simulink model "simulation_pv_parallel"  (R2020b)
settings: Solver=FixedStepAuto  StartTime=0.0  StopTime=sim_length  FixedStep=1  RelTol=1e-3
values from neighbouring files (symbols this model uses):
  air_delay = 0    [analysis.m]    (also in config.m; matlab.mat; workspace.mat)
  air_pulse = (air_time * 100)/period    [analysis.m]    (also in config.m = 25; matlab.mat = 25; workspace.mat = 25)
  efficiency_pv = [0.0206 0.0224 0.0235 0.0258 0.0287 0.0304 0.0361 0.0396 0.0436 0.047 0.0774 0.0866 ... (52 elements, 26x2)]    [matlab.mat]    (also in workspace.mat)
  efficiencybatterydcdc = [0.0136458313659 0.015570408259 0.019337485453 0.0242437613353 0.0298263424578 0.0373938343643 0.0491473380199 0.0560789663375 0.0670656286702 0.0809654995908 0.0941455940195 0.113657997475 ... (56 elements, 28x2)]    [workspace.mat]
  G = [250;500;750;1000]    [lab3_day1.m]    (also in matlab.mat = [250 500 750 1000]; workspace.mat = [250 500 750 1000])
  I = [Impp_250;Impp_500;Impp_750;Impp_1000]    [lab3_day1.m]    (also in matlab.mat = [0.01272 0.02816 0.04153 0.05463]; workspace.mat = [0.01272 0.02816 0.04153 0.05463])
  mc_delay = mic_delay + mic_time    [analysis.m]    (also in config.m = 30; matlab.mat = 30; workspace.mat = 30)
  mc_pulse = (mc_time*100)/period    [analysis.m]    (also in config.m = 5; matlab.mat = 5; workspace.mat = 5)
  methane_delay = air_time    [analysis.m]    (also in config.m = 0; matlab.mat = 0; workspace.mat = 0)
  methane_pulse = (methane_time * 100)/period    [analysis.m]    (also in config.m = 25; matlab.mat = 25; workspace.mat = 25)
  mic_delay = temp_delay + temp_time    [analysis.m]    (also in config.m = 0; matlab.mat = 0; workspace.mat = 0)
  mic_pulse = (mic_time * 100)/period    [analysis.m]    (also in config.m = 10; matlab.mat = 10; workspace.mat = 10)
  period = 240    [analysis.m]    (also in config.m = 120; matlab.mat = 120; workspace.mat = 120)
  temp_delay = methane_delay + methane_time    [analysis.m]    (also in config.m = 0; matlab.mat = 0; workspace.mat = 0)
  temp_pulse = (temp_time *100)/period    [analysis.m]    (also in config.m = 5; matlab.mat = 5; workspace.mat = 5)
  transmit_delay = mc_delay + mc_time    [analysis.m]    (also in config.m = 36; matlab.mat = 36; workspace.mat = 36)
  transmit_pulse = (transmit_time * 100)/period    [analysis.m]    (also in config.m = 20; matlab.mat = 20; workspace.mat = 20)
  V = [Vmpp_250;Vmpp_500;Vmpp_750;Vmpp_1000]    [lab3_day1.m]    (also in matlab.mat = [3.1 3.14 3.15 3.3]; workspace.mat = [3.1 3.14 3.15 3.3])
libraries: simulink x10
settings Model: Creator=sara  LastModifiedBy=Nicolò
settings DataIOCC: ReturnWorkspaceOutputs=off
settings DebuggingCC: ArithmeticOperatorsInVariantConditions=warning
settings SFSimCC: SimUseLocalCustomCode=off  CustomCodeUndefinedFunction=UseInterfaceOnly
settings RTWCC: RTWUseLocalCustomCode=off
settings CodeAppCC: StateflowObjectComments=on

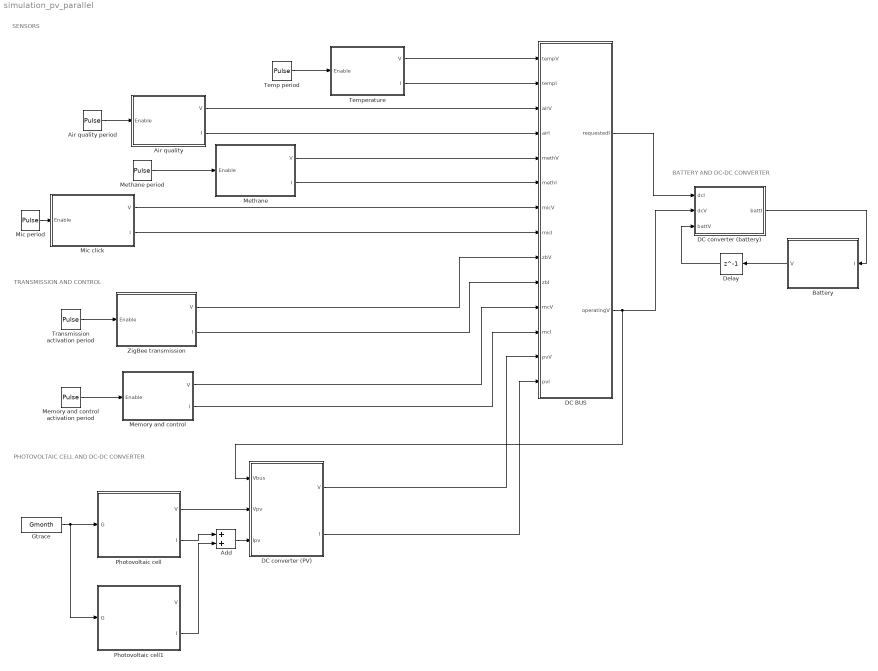
== system simulation_pv_parallel ==
  note: TRANSMISSION AND CONTROL
  note: SENSORS
  note: PHOTOVOLTAIC CELL AND DC-DC CONVERTER
  note: BATTERY AND DC-DC CONVERTER
  Add : Sum
  Air quality : Subsystem
  Air quality period : DiscretePulseGenerator  PulseType=Time based  Period=period  PulseWidth=air_pulse  PhaseDelay=air_delay
  Battery : Subsystem
  DC BUS : Subsystem
  DC converter (PV) : Subsystem
  DC converter (battery) : Subsystem
  Delay : Delay  DelayLength=1  InitialCondition=0
  Gtrace : FromWorkspace  VariableName=Gmonth  OutputAfterFinalValue=Setting to zero
  Memory and control : Subsystem
  Memory and control activation period : DiscretePulseGenerator  PulseType=Time based  Period=period  PulseWidth=mc_pulse  PhaseDelay=mc_delay
  Methane : Subsystem
  Methane period : DiscretePulseGenerator  PulseType=Time based  Period=period  PulseWidth=methane_pulse  PhaseDelay=methane_delay
  Mic period : DiscretePulseGenerator  PulseType=Time based  Period=period  PulseWidth=mic_pulse  PhaseDelay=mic_delay
  Mic click : Subsystem
  Photovoltaic cell : Subsystem
  Photovoltaic cell1 : Subsystem
  Temp period : DiscretePulseGenerator  PulseType=Time based  Period=period  PulseWidth=temp_pulse  PhaseDelay=temp_delay
  Temperature : Subsystem
  Transmission activation period : DiscretePulseGenerator  PulseType=Time based  Period=period  PulseWidth=transmit_pulse  PhaseDelay=transmit_delay
  ZigBee transmission : Subsystem
  wires:
  Gtrace/1 -> Photovoltaic cell1/1(G), Photovoltaic cell/1(G)
  Mic click/2(I) -> DC BUS/8(micI)
  Mic click/1(V) -> DC BUS/7(micV)
  Mic period/1 -> Mic click/1(Enable)
  Air quality period/1 -> Air quality/1(Enable)
  Air quality/1(V) -> DC BUS/3(airV)
  Air quality/2(I) -> DC BUS/4(airI)
  Methane/1(V) -> DC BUS/5(methV)
  Methane period/1 -> Methane/1(Enable)
  Methane/2(I) -> DC BUS/6(methI)
  Temperature/1(V) -> DC BUS/1(tempV)
  Temp period/1 -> Temperature/1(Enable)
  ZigBee transmission/1(V) -> DC BUS/9(zbV)
  Transmission activation period/1 -> ZigBee transmission/1(Enable)
  Temperature/2(I) -> DC BUS/2(tempI)
  Memory and control/1(V) -> DC BUS/11(mcV)
  ZigBee transmission/2(I) -> DC BUS/10(zbI)
  Battery/1(V) -> Delay/1
  DC converter (battery)/1(battI) -> Battery/1(I)
  DC BUS/1(requestedI) -> DC converter (battery)/1(dcI)
  DC BUS/2(operatingV) -> DC converter (PV)/1(Vbus), DC converter (battery)/2(dcV)
  Delay/1 -> DC converter (battery)/3(battV)
  DC converter (PV)/2(I) -> DC BUS/14(pvI)
  DC converter (PV)/1(V) -> DC BUS/13(pvV)
  Memory and control/2(I) -> DC BUS/12(mcI)
  Memory and control activation period/1 -> Memory and control/1(Enable)
  Add/1 -> DC converter (PV)/3(Ipv)
  Photovoltaic cell/2(I) -> Add/1
  Photovoltaic cell1/2(I) -> Add/2
  Photovoltaic cell/1(V) -> DC converter (PV)/2(Vpv)

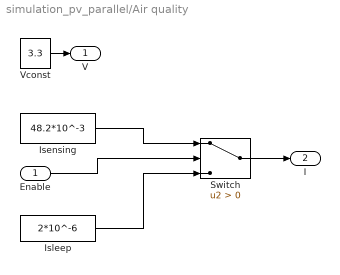
== system simulation_pv_parallel/Air quality ==
  Enable : Inport
  Isensing : Constant  Value=48.2*10^-3
  Isleep : Constant  Value=2*10^-6
  Switch : Switch  Criteria=u2 > Threshold
  Vconst : Constant  Value=3.3
  V : Outport
  I : Outport  Port=2
  wires:
  Enable/1 -> Switch/2
  Isleep/1 -> Switch/3
  Vconst/1 -> V/1
  Isensing/1 -> Switch/1
  Switch/1 -> I/1

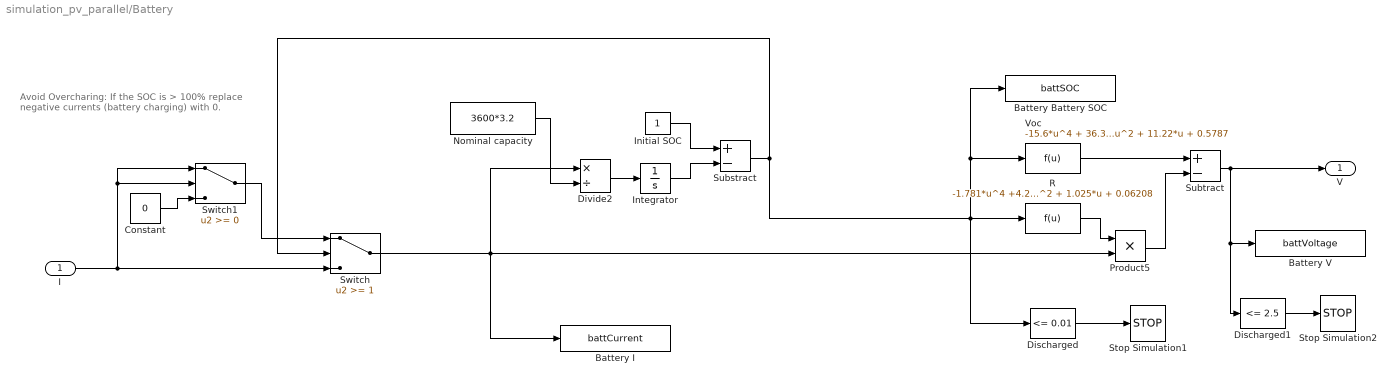
== system simulation_pv_parallel/Battery ==
  note: Avoid Overcharing:
      | If the SOC is > 100% replace negative currents (battery charging) with 0.
  I : Inport
  Battery Battery SOC : ToWorkspace  VariableName=battSOC  SampleTime=-1
  Battery I : ToWorkspace  VariableName=battCurrent  SampleTime=-1
  Battery V : ToWorkspace  VariableName=battVoltage  SampleTime=-1
  Constant : Constant  Value=0
  Discharged : simulink/Logic and Bit Operations/Compare To Constant  relop=<=  const=0.01  OutDataTypeStr=boolean  ZeroCross=off
  Discharged1 : simulink/Logic and Bit Operations/Compare To Constant  relop=<=  const=2.5  OutDataTypeStr=boolean  ZeroCross=off
  Divide2 : Product  Inputs=*/
  Initial SOC : Constant
  Integrator : Integrator
  Nominal capacity : Constant  Value=3600*3.2
  Product5 : Product  RndMeth=Zero
  R : Fcn  Expr=-1.781*u^4 +4.222*u^3 -3.401*u^2 + 1.025*u + 0.06208
  Stop Simulation1 : Stop
  Stop Simulation2 : Stop
  Substract : Sum  Inputs=+-
  Subtract : Sum  Inputs=+-
  Switch : Switch  Threshold=1
  Switch1 : Switch
  Voc : Fcn  Expr=-15.6*u^4 + 36.33*u^3 - 29.04*u^2 + 11.22*u + 0.5787
  V : Outport
  wires:
  Integrator/1 -> Substract/2
  Nominal capacity/1 -> Divide2/2
  Divide2/1 -> Integrator/1
  Voc/1 -> Subtract/1
  Subtract/1 -> Battery V/1, Discharged1/1, V/1
  I/1 -> Switch/3, Switch1/1, Switch1/2
  Product5/1 -> Subtract/2
  R/1 -> Product5/1
  Discharged/1 -> Stop Simulation1/1
  Initial SOC/1 -> Substract/1
  Discharged1/1 -> Stop Simulation2/1
  Substract/1 -> Voc/1, Battery Battery SOC/1, Discharged/1, R/1, Switch/2
  Switch/1 -> Divide2/1, Product5/2, Battery I/1
  Switch1/1 -> Switch/1
  Constant/1 -> Switch1/3

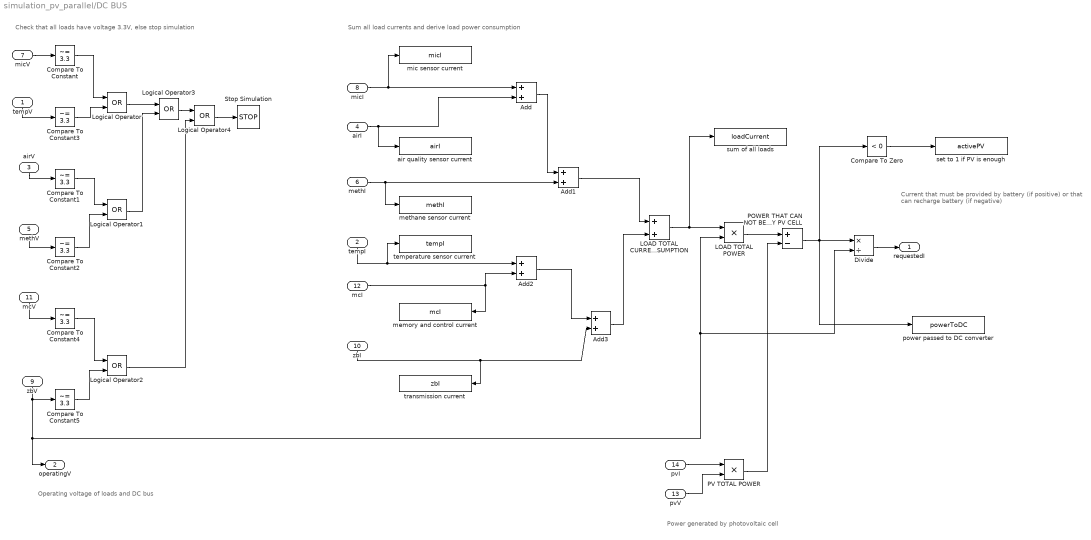
== system simulation_pv_parallel/DC BUS ==
  note: Check that all loads have voltage 3.3V, else stop simulation
  note: Sum all load currents and derive load power consumption
  note: Power generated by photovoltaic cell
  note: Current that must be provided by battery (if positive) or that can recharge battery (if negative)
  note: Operating voltage of loads and DC bus
  tempV : Inport
  tempI : Inport  Port=2
  airV : Inport  Port=3
  airI : Inport  Port=4
  methV : Inport  Port=5
  methI : Inport  Port=6
  micV : Inport  Port=7
  micI : Inport  Port=8
  zbV : Inport  Port=9
  zbI : Inport  Port=10
  mcV : Inport  Port=11
  mcI : Inport  Port=12
  pvV : Inport  Port=13
  pvI : Inport  Port=14
  Add{,1..3} (4 alike) : Sum
  Compare To Constant{,1..5} (6 alike) : simulink/Logic and Bit Operations/Compare To Constant  relop=~=  const=3.3  OutDataTypeStr=boolean
  Compare To Zero : simulink/Logic and Bit Operations/Compare To Zero  relop=<  OutDataTypeStr=boolean
  Divide : Product  Inputs=*/
  LOAD TOTAL CURRENT CONSUMPTION : Sum
  LOAD TOTAL POWER : Product
  Logical Operator{,1..4} (5 alike) : Logic  Operator=OR  AllPortsSameDT=off  OutDataTypeStr=boolean
  POWER THAT CAN NOT BE PROVIDED BY PV CELL : Sum  Inputs=+-
  PV TOTAL POWER : Product
  Stop Simulation : Stop
  air quality sensor current : ToWorkspace  VariableName=airI  SampleTime=-1
  memory and control current : ToWorkspace  VariableName=mcI  SampleTime=-1
  methane sensor current : ToWorkspace  VariableName=methI  SampleTime=-1
  mic sensor current : ToWorkspace  VariableName=micI  SampleTime=-1
  power passed to DC converter : ToWorkspace  VariableName=powerToDC  SampleTime=-1
  set to 1 if PV is enough : ToWorkspace  VariableName=activePV  SampleTime=-1
  sum of all loads : ToWorkspace  VariableName=loadCurrent  SampleTime=-1
  temperature sensor current : ToWorkspace  VariableName=tempI  SampleTime=-1
  transmission current : ToWorkspace  VariableName=zbI  SampleTime=-1
  requestedI : Outport
  operatingV : Outport  Port=2
  wires:
  airV/1 -> Compare To Constant1/1
  Add/1 -> Add1/1
  zbV/1 -> operatingV/1, Divide/2, LOAD TOTAL POWER/2, Compare To Constant5/1
  methI/1 -> methane sensor current/1, Add1/2
  methV/1 -> Compare To Constant2/1
  micV/1 -> Compare To Constant/1
  micI/1 -> mic sensor current/1, Add/1
  mcV/1 -> Compare To Constant4/1
  Add3/1 -> LOAD TOTAL CURRENT CONSUMPTION/2
  airI/1 -> air quality sensor current/1, Add/2
  Add1/1 -> LOAD TOTAL CURRENT CONSUMPTION/1
  tempV/1 -> Compare To Constant3/1
  Compare To Constant/1 -> Logical Operator/1
  Compare To Constant3/1 -> Logical Operator/2
  Compare To Constant1/1 -> Logical Operator1/1
  Compare To Constant2/1 -> Logical Operator1/2
  Compare To Constant4/1 -> Logical Operator2/1
  Compare To Constant5/1 -> Logical Operator2/2
  Logical Operator/1 -> Logical Operator3/1
  Logical Operator1/1 -> Logical Operator3/2
  Logical Operator3/1 -> Logical Operator4/1
  Logical Operator2/1 -> Logical Operator4/2
  Logical Operator4/1 -> Stop Simulation/1
  mcI/1 -> Add2/2, memory and control current/1
  tempI/1 -> temperature sensor current/1, Add2/1
  Add2/1 -> Add3/1
  zbI/1 -> transmission current/1, Add3/2
  pvI/1 -> PV TOTAL POWER/1
  pvV/1 -> PV TOTAL POWER/2
  LOAD TOTAL CURRENT CONSUMPTION/1 -> sum of all loads/1, LOAD TOTAL POWER/1
  LOAD TOTAL POWER/1 -> POWER THAT CAN NOT BE PROVIDED BY PV CELL/1
  PV TOTAL POWER/1 -> POWER THAT CAN NOT BE PROVIDED BY PV CELL/2
  POWER THAT CAN NOT BE PROVIDED BY PV CELL/1 -> power passed to DC converter/1, Compare To Zero/1, Divide/1
  Divide/1 -> requestedI/1
  Compare To Zero/1 -> set to 1 if PV is enough/1

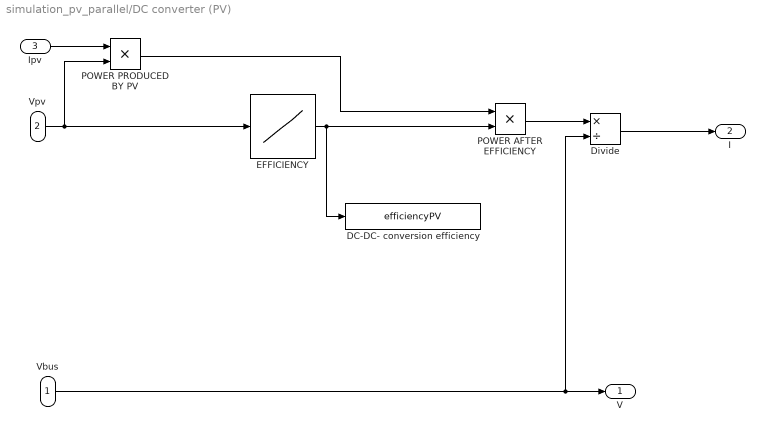
== system simulation_pv_parallel/DC converter (PV) ==
  Vbus : Inport
  Vpv : Inport  Port=2
  Ipv : Inport  Port=3
  DC-DC- conversion efficiency : ToWorkspace  VariableName=efficiencyPV  SampleTime=-1
  Divide : Product  Inputs=*/
  EFFICIENCY : Lookup_n-D  NumberOfTableDimensions=1  BreakpointsForDimension1=efficiency_pv(:,1)  Table=efficiency_pv(:,2)  InternalRulePriority=Speed  RndMeth=Simplest  InputSameDT=on
  POWER PRODUCED BY PV : Product
  "POWER AFTER EFFICIENCY " : Product
  V : Outport
  I : Outport  Port=2
  wires:
  "POWER AFTER EFFICIENCY "/1 -> Divide/1
  Vbus/1 -> Divide/2, V/1
  POWER PRODUCED BY PV/1 -> "POWER AFTER EFFICIENCY "/1
  Divide/1 -> I/1
  EFFICIENCY/1 -> DC-DC- conversion efficiency/1, "POWER AFTER EFFICIENCY "/2
  Ipv/1 -> POWER PRODUCED BY PV/1
  Vpv/1 -> POWER PRODUCED BY PV/2, EFFICIENCY/1

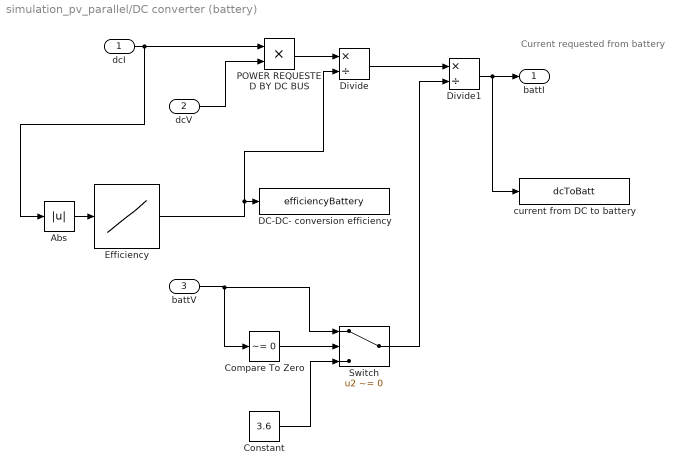
== system simulation_pv_parallel/DC converter (battery) ==
  note: Current requested from battery
  dcI : Inport
  dcV : Inport  Port=2
  battV : Inport  Port=3
  Abs : Abs
  Compare To Zero : simulink/Logic and Bit Operations/Compare To Zero  relop=~=  OutDataTypeStr=boolean
  Constant : Constant  Value=3.6
  DC-DC- conversion efficiency : ToWorkspace  VariableName=efficiencyBattery  SampleTime=-1
  Divide : Product  Inputs=*/
  Divide1 : Product  Inputs=*/
  Efficiency : Lookup_n-D  NumberOfTableDimensions=1  BreakpointsForDimension1=efficiencybatterydcdc(:,1)  Table=efficiencybatterydcdc(:,2)  InternalRulePriority=Speed  RndMeth=Simplest  InputSameDT=on
  POWER REQUESTED BY DC BUS : Product
  Switch : Switch  Criteria=u2 ~= 0
  current from DC to battery : ToWorkspace  VariableName=dcToBatt  SampleTime=-1
  battI : Outport
  wires:
  dcV/1 -> POWER REQUESTED BY DC BUS/2
  POWER REQUESTED BY DC BUS/1 -> Divide/1
  Divide/1 -> Divide1/1
  Divide1/1 -> current from DC to battery/1, battI/1
  dcI/1 -> Abs/1, POWER REQUESTED BY DC BUS/1
  battV/1 -> Switch/1, Compare To Zero/1
  Compare To Zero/1 -> Switch/2
  Constant/1 -> Switch/3
  Switch/1 -> Divide1/2
  Efficiency/1 -> Divide/2, DC-DC- conversion efficiency/1
  Abs/1 -> Efficiency/1

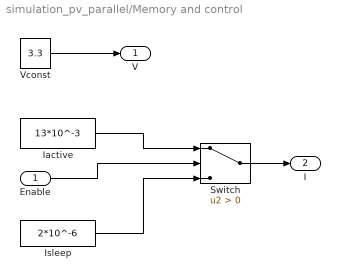
== system simulation_pv_parallel/Memory and control ==
  Enable : Inport
  Iactive : Constant  Value=13*10^-3
  Isleep : Constant  Value=2*10^-6
  Switch : Switch  Criteria=u2 > Threshold
  Vconst : Constant  Value=3.3
  V : Outport
  I : Outport  Port=2
  wires:
  Vconst/1 -> V/1
  Iactive/1 -> Switch/1
  Switch/1 -> I/1
  Isleep/1 -> Switch/3
  Enable/1 -> Switch/2

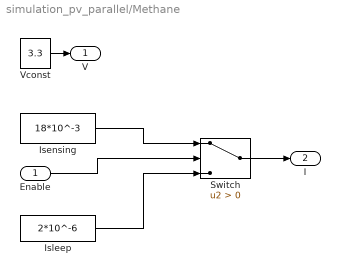
== system simulation_pv_parallel/Methane ==
  Enable : Inport
  Isensing : Constant  Value=18*10^-3
  Isleep : Constant  Value=2*10^-6
  Switch : Switch  Criteria=u2 > Threshold
  Vconst : Constant  Value=3.3
  V : Outport
  I : Outport  Port=2
  wires:
  Enable/1 -> Switch/2
  Isleep/1 -> Switch/3
  Vconst/1 -> V/1
  Isensing/1 -> Switch/1
  Switch/1 -> I/1

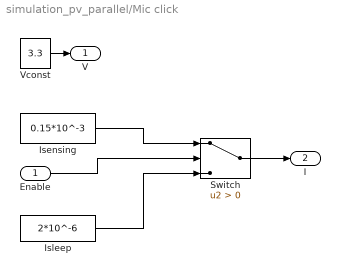
== system simulation_pv_parallel/Mic click ==
  Enable : Inport
  Isensing : Constant  Value=0.15*10^-3
  Isleep : Constant  Value=2*10^-6
  Switch : Switch  Criteria=u2 > Threshold
  Vconst : Constant  Value=3.3
  V : Outport
  I : Outport  Port=2
  wires:
  Enable/1 -> Switch/2
  Isleep/1 -> Switch/3
  Vconst/1 -> V/1
  Isensing/1 -> Switch/1
  Switch/1 -> I/1

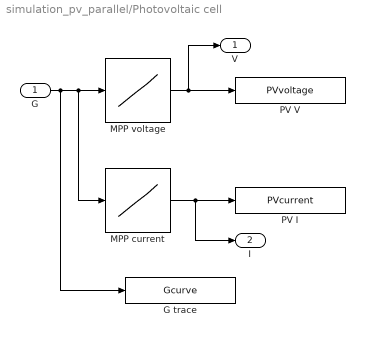
== system simulation_pv_parallel/Photovoltaic cell ==
  G : Inport
  G trace : ToWorkspace  VariableName=Gcurve  SampleTime=-1
  MPP current : Lookup_n-D  NumberOfTableDimensions=1  BreakpointsForDimension1=G  Table=I  InternalRulePriority=Speed  RndMeth=Simplest  InputSameDT=on
  MPP voltage : Lookup_n-D  NumberOfTableDimensions=1  BreakpointsForDimension1=G  Table=V  InternalRulePriority=Speed  RndMeth=Simplest  InputSameDT=on
  PV I : ToWorkspace  VariableName=PVcurrent  SampleTime=-1
  PV V : ToWorkspace  VariableName=PVvoltage  SampleTime=-1
  V : Outport
  I : Outport  Port=2
  wires:
  MPP voltage/1 -> PV V/1, V/1
  MPP current/1 -> PV I/1, I/1
  G/1 -> G trace/1, MPP current/1, MPP voltage/1

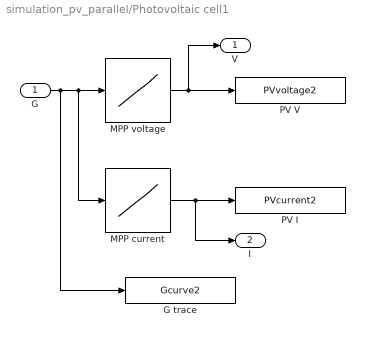
== system simulation_pv_parallel/Photovoltaic cell1 ==
  G : Inport
  G trace : ToWorkspace  VariableName=Gcurve2  SampleTime=-1
  MPP current : Lookup_n-D  NumberOfTableDimensions=1  BreakpointsForDimension1=G  Table=I  InternalRulePriority=Speed  RndMeth=Simplest  InputSameDT=on
  MPP voltage : Lookup_n-D  NumberOfTableDimensions=1  BreakpointsForDimension1=G  Table=V  InternalRulePriority=Speed  RndMeth=Simplest  InputSameDT=on
  PV I : ToWorkspace  VariableName=PVcurrent2  SampleTime=-1
  PV V : ToWorkspace  VariableName=PVvoltage2  SampleTime=-1
  V : Outport
  I : Outport  Port=2
  wires:
  MPP voltage/1 -> PV V/1, V/1
  MPP current/1 -> PV I/1, I/1
  G/1 -> G trace/1, MPP current/1, MPP voltage/1

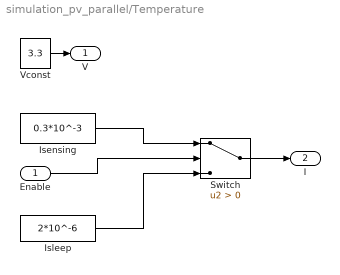
== system simulation_pv_parallel/Temperature ==
  Enable : Inport
  Isensing : Constant  Value=0.3*10^-3
  Isleep : Constant  Value=2*10^-6
  Switch : Switch  Criteria=u2 > Threshold
  Vconst : Constant  Value=3.3
  V : Outport
  I : Outport  Port=2
  wires:
  Enable/1 -> Switch/2
  Isleep/1 -> Switch/3
  Vconst/1 -> V/1
  Isensing/1 -> Switch/1
  Switch/1 -> I/1

== system simulation_pv_parallel/ZigBee transmission ==
  Enable : Inport
  Iidle : Constant  Value=1*10^-6
  Itransmitting : Constant  Value=0.1*10^-3
  Switch : Switch  Criteria=u2 > Threshold
  Vconst : Constant  Value=3.3
  V : Outport
  I : Outport  Port=2
  wires:
  Enable/1 -> Switch/2
  Iidle/1 -> Switch/3
  Vconst/1 -> V/1
  Itransmitting/1 -> Switch/1
  Switch/1 -> I/1
